simulink model "pdcontroller"  (R2025b)
settings: Solver=ode113  StartTime=0.0  StopTime=30*60  RelTol=1e-3
undefined symbols (not defined in the file): params, q0, r_start, v_start, w0
settings Model: Creator=alexanderkavetsky  LastModifiedBy=alexanderkavetsky

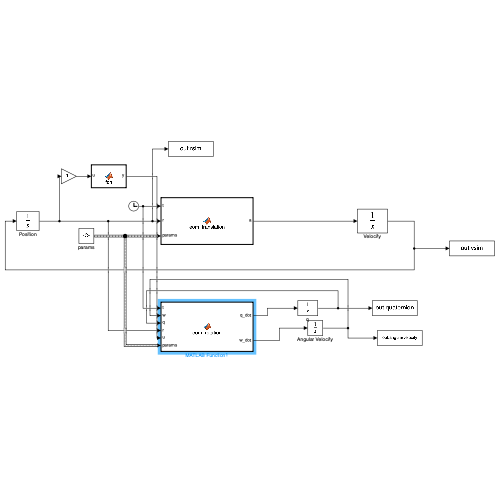
[thumbnail: Simulink's stored preview of the top-level diagram]
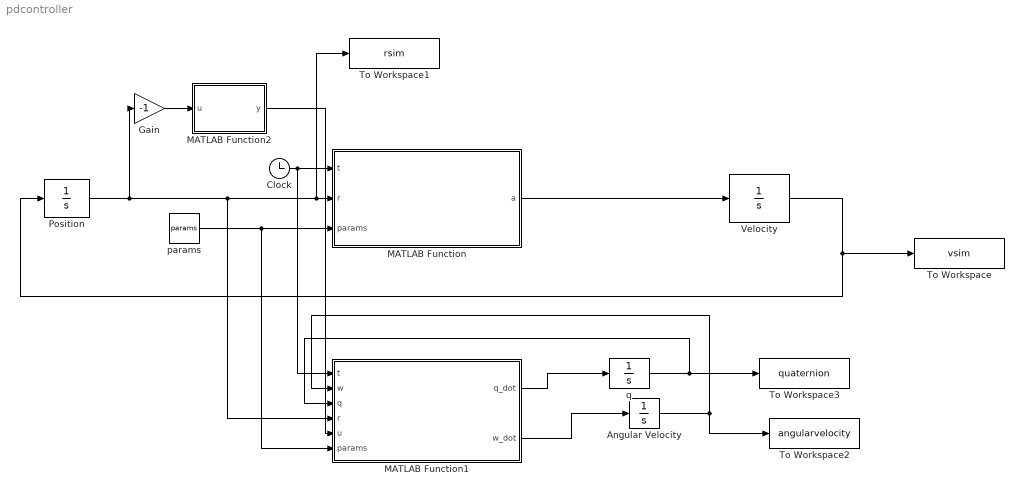
== system pdcontroller ==
  Angular Velocity : Integrator  InitialCondition=w0
  Clock : Clock
  Gain : Gain  Gain=-1
  MATLAB Function : MATLAB Function  TreatAsAtomicUnit=on
  MATLAB Function1 : MATLAB Function  TreatAsAtomicUnit=on
  MATLAB Function2 : MATLAB Function  TreatAsAtomicUnit=on
  Position : Integrator  InitialCondition=r_start
  To Workspace : ToWorkspace  VariableName=vsim  SampleTime=-1
  To Workspace1 : ToWorkspace  VariableName=rsim  SampleTime=-1
  To Workspace2 : ToWorkspace  VariableName=angularvelocity  SaveFormat=Timeseries  SampleTime=-1
  To Workspace3 : ToWorkspace  VariableName=quaternion  SaveFormat=Timeseries  SampleTime=-1
  Velocity : Integrator  InitialCondition=v_start
  params : Constant  Value=params  OutDataTypeStr=Bus: slBus1  LockScale=on
  q : Integrator  InitialCondition=q0
  wires:
  Velocity/1 -> Position/1, To Workspace/1
  MATLAB Function/1(a) -> Velocity/1
  Angular Velocity/1 -> To Workspace2/1, MATLAB Function1/2(w)
  Clock/1 -> MATLAB Function1/1(t), MATLAB Function/1(t)
  MATLAB Function1/2(w_dot) -> Angular Velocity/1
  q/1 -> To Workspace3/1, MATLAB Function1/3(q)
  Position/1 -> Gain/1, MATLAB Function/2(r), To Workspace1/1, MATLAB Function1/4(r)
  MATLAB Function1/1(q_dot) -> q/1
  params/1 -> MATLAB Function1/6(params), MATLAB Function/3(params)
  Gain/1 -> MATLAB Function2/1(u)
  MATLAB Function2/1(y) -> MATLAB Function1/5(u)

== matlab function pdcontroller/MATLAB Function1 ==
  data: t input; q_dot output; w input; q input; r input; u input; params input; w_dot output
function [q_dot, w_dot] = eom_rotation(t,w,q,r,u,params)
I = params.I; 
% Calculate torques 
tau = torque(r, q, params); 
u_quat = quat_rotate(q, u); 
v_panel_body = [0;  0; 1 ]; 
error = cross(v_panel_body, u_quat); 

% Define Gains for PD Controller 
Kp = 0.01; 
Kd = 2.4; 

% Calculate torques
torque_control = -(Kp * error) - (Kd * w); 
torque_total = tau + torque_control;
% Normalize q to prevent drift 
q = q / norm(q); 
q_dot = 0.5 * omega_matrix(w) * q;
w_dot = I \ (torque_total - cross(w, I * w));
end

== matlab function pdcontroller/MATLAB Function ==
  data: t input; r input; a output; params input
function a = eom_translation(t,r,params)
    % Calculating two body acceleration 
    a_twobody = -params.MUSun/norm(r)^3 * r;
    jupiter = propagate_elliptical(params.jup_200, t, params.MUSun);
    % Calculating acceleration for third body
    ajupiter = thirdbody(params.MUJup, r, jupiter(1:3));
    % Calculating acceleration due to srp 
    a_srp = srp(r*1000, params)/1000; 
    % Adding up accerlerations for equations of motion 
    a = a_twobody + ajupiter + a_srp; 
end

== matlab function pdcontroller/MATLAB Function2 ==
  data: u input; y output
function y = fcn(u)

norm_u = norm(u); 
y = u/norm_u;
